simulink model "Mass_outflow"  (R2024b)
settings: Solver=ode45  StartTime=0.0  StopTime=10.0  RelTol=1e-3
settings Model: Creator=viviankaspar  LastModifiedBy=viviankaspar

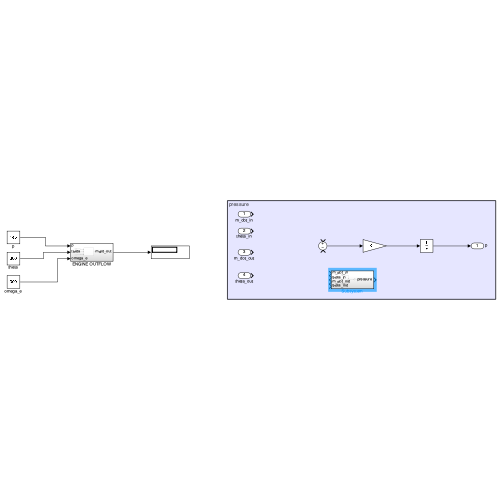
[thumbnail: Simulink's stored preview of the top-level diagram]
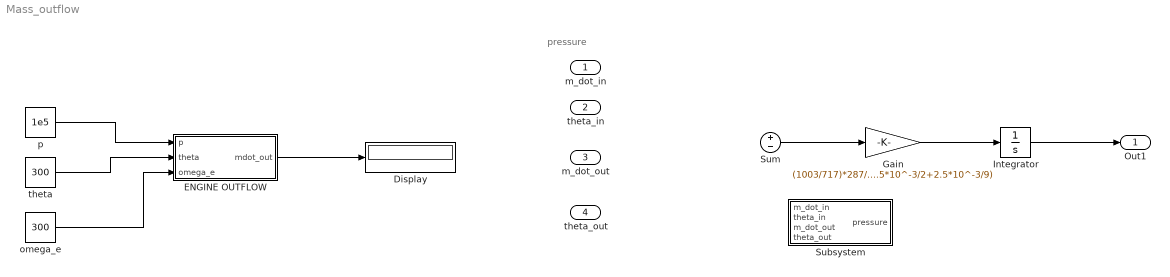
== system Mass_outflow ==
  note: pressure
  m_dot_in : Inport
  theta_in : Inport  Port=2
  m_dot_out : Inport  Port=3
  theta_out : Inport  Port=4
  Display : Display
  ENGINE OUTFLOW : Subsystem
  Gain : Gain  Gain=(1003/717)*287/(2.5*10^-3/2+2.5*10^-3/9)  mask{kappa=1003/717, R=287, Vd=2.5*10^-3, epsilon=10}
  Integrator : Integrator  InitialCondition=10^5
  Subsystem : Subsystem
  Sum : Sum  Inputs=+-
  omega_e : Constant  Value=300
  p : Constant  Value=1e5
  theta : Constant  Value=300
  Out1 : Outport  SignalName=p
  wires:
  p/1 -> ENGINE OUTFLOW/1(p)
  theta/1 -> ENGINE OUTFLOW/2(theta)
  omega_e/1 -> ENGINE OUTFLOW/3(omega_e)
  ENGINE OUTFLOW/1(mdot_out) -> Display/1
  Sum/1 -> Gain/1
  Gain/1 -> Integrator/1
  Integrator/1 -> Out1/1

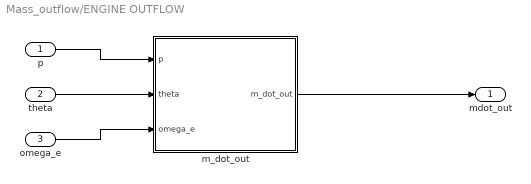
== system Mass_outflow/ENGINE OUTFLOW ==
  p : Inport
  theta : Inport  Port=2
  omega_e : Inport  Port=3
  m_dot_out : MATLAB Function  TreatAsAtomicUnit=on  mask{Vd=2.5*10^-3, kappa=1003/717, R=287, epsilon=10, pe=10^5, lambda_lw=0.8}
  mdot_out : Outport
  wires:
  p/1 -> m_dot_out/1(p)
  theta/1 -> m_dot_out/2(theta)
  omega_e/1 -> m_dot_out/3(omega_e)
  m_dot_out/1(m_dot_out) -> mdot_out/1

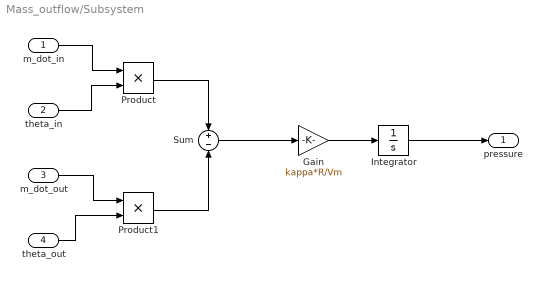
== system Mass_outflow/Subsystem ==
  m_dot_in : Inport
  theta_in : Inport  Port=2
  m_dot_out : Inport  Port=3
  theta_out : Inport  Port=4
  Gain : Gain  Gain=kappa*R/Vm  mask{kappa=1003/717, R=287, Vm=2.5*10^-3*(1/2+1/9)}
  Integrator : Integrator  InitialCondition=10^5  LimitOutput=on  UpperSaturationLimit=5e6
  Product : Product
  Product1 : Product
  Sum : Sum  Inputs=+-
  pressure : Outport
  wires:
  m_dot_in/1 -> Product/1
  theta_in/1 -> Product/2
  m_dot_out/1 -> Product1/1
  theta_out/1 -> Product1/2
  Product/1 -> Sum/1
  Product1/1 -> Sum/2
  Sum/1 -> Gain/1
  Gain/1 -> Integrator/1
  Integrator/1 -> pressure/1

== matlab function Mass_outflow/ENGINE OUTFLOW/m_dot_out ==
  data: p input; m_dot_out output; theta input; omega_e input; Vd parameter; kappa parameter; R parameter; pe parameter; lambda_lw parameter; epsilon parameter
function m_dot_out = fcn(p,theta,omega_e, Vd, kappa, R, pe, lambda_lw, epsilon)

m_dot_out = p/(R*theta)*Vd*omega_e/(4*pi)*lambda_lw*(epsilon/(epsilon-1)-1/(epsilon-1)*(pe/p)^(1/kappa));
